simulink model "q10"  (R2017b)
settings: Solver=VariableStepAuto  StartTime=0.0  StopTime=3  RelTol=1e-3
undefined symbols (not defined in the file): Az, Bz, K
settings Model: Creator=admin  LastModifiedBy=admin

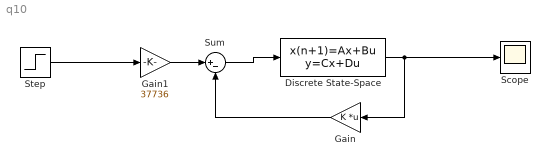
== system q10 ==
  Discrete State-Space : DiscreteStateSpace  A=Az  B=Bz  C=eye(3)  D=[0;0;0]  SampleTime=0.004
  Gain : Gain  Gain=K  Multiplication=Matrix(K*u)
  Gain1 : Gain  Gain=37736
  Scope : Scope
  Step : Step  SampleTime=0
  Sum : Sum  Inputs=|+-
  wires:
  Discrete State-Space/1 -> Scope/1, Gain/1
  Gain/1 -> Sum/2
  Sum/1 -> Discrete State-Space/1
  Gain1/1 -> Sum/1
  Step/1 -> Gain1/1
